simulink model "HANcoder_E407_Matrix"  (R2018b)
settings: Solver=FixedStepDiscrete  StartTime=0.0  StopTime=1  FixedStep=0.01  RelTol=1e-3
PreLoadFcn:
  | librarySetup
  | eval([bdroot,'_startup']) %Calling [modelName]_startup.m
undefined symbols (not defined in the file): frequency_IRQ, HANtuneOverride, idle_time, LED_ticks_toggle
libraries: HANcoder_STM32_Target x15, simulink x6, simulink_extras x1
CloseFcn:
  | rtwprivate ssgencode ModelCloseRequest mytest
settings Model: Creator=Jason van Kolfschoten  LastModifiedBy=Jamie
settings SolverCC: PositivePriorityOrder=on
settings DataIOCC: LimitDataPoints=on  SaveFormat=Array  SignalLoggingSaveFormat=ModelDataLogs  SaveOutput=off  SaveTime=off
settings OptimizationCC: BlockReduction=off  DefaultParameterBehavior=Inlined  InlineInvariantSignals=on  ExpressionDepthLimit=2147483647  StateBitsets=on  DataBitsets=on  ZeroExternalMemoryAtStartup=off  ZeroInternalMemoryAtStartup=off  InitFltsAndDblsToZero=on  NoFixptDivByZeroProtection=on  EfficientFloat2IntCast=on  LifeSpan=inf
settings DebuggingCC: SaveWithDisabledLinksMsg=none  SaveWithParameterizedLinksMsg=none  CheckSSInitialOutputMsg=off  UnderspecifiedInitializationDetection=Classic  MergeDetectMultiDrivingBlocksExec=none  SignalResolutionControl=TryResolveAll  SolverPrmCheckMsg=warning  InheritedTsInSrcMsg=none  MultiTaskDSMMsg=warning  MultiTaskCondExecSysMsg=none  ParameterPrecisionLossMsg=none  FcnCallInpInsideContextMsg=warning  StateNameClashWarn=warning  SFUnexpectedBacktrackingDiag=warning  SFNoUnconditionalDefaultTransitionDiag=warning  SFExecutionAtInitializationDiag=none
settings HardwareCC: ProdBitPerPointer=32  ProdBitPerSizeT=32  ProdBitPerPtrDiffT=32  ProdLargestAtomicFloat=None  ProdIntDivRoundTo=Undefined  ProdWordSize=32  ProdHWDeviceType=Generic->32-bit Embedded Processor  TargetEndianess=LittleEndian  TargetHWDeviceType=Infineon->TriCore
settings ModelReferenceCC: PropagateSignalLabelsOutOfModel=off
settings SFSimCC: SimUseLocalCustomCode=off  MATLABDynamicMemAlloc=off
settings RTWCC: SystemTargetFile=ert.tlc  MakeCommand=make_rtw SHELL= HANcoder_PORTABLE=1 HANcoder_BOOTLOADER=1  TemplateMakefile=STM32_E407_gcc.tmf  Description=Real-Time Workshop Embedded Coder (no auto configuration)  RTWUseLocalCustomCode=off
settings CodeAppCC: ForceParamTrailComments=on  IgnoreCustomStorageClasses=off  SimulinkDataObjDesc=on  CustomSymbolStrGlobalVar=rt$N$M  CustomSymbolStrType=$N$M  CustomSymbolStrFcn=$N$M$F  CustomSymbolStrMacro=$N$M  InsertBlockDesc=on  StateflowObjectComments=on  InternalIdentifier=Classic
settings ERTTargetCC: TargetFcnLib=ansi_tfl_tmw.mat  MultiwordLength=2048  IncludeMdlTerminateFcn=off  SuppressErrorStatus=on  SupportNonFinite=off  GenerateASAP2=on  InlinedParameterPlacement=NonHierarchical  ERTCustomFileTemplate=example_file_process.tlc  ConvertIfToSwitch=off  SuppressUnreachableDefaultCases=off
settings ConfigComp: CovMetricSettings=dw  CovHtmlReporting=on  CovSaveCumulativeToWorkspaceVar=on  CovSaveSingleToWorkspaceVar=on  CovExternalEMLEnable=off  DVMaxProcessTime=600  DVDisplayUnsatisfiableObjectives=on  DVAutomaticStubbing=off  DVModelCoverageObjectives=MCDC  DVMaxTestCaseSteps=500  DVTestSuiteOptimization=CombinedObjectives  DVDetectActiveLogic=on  DVSaveHarnessModel=on

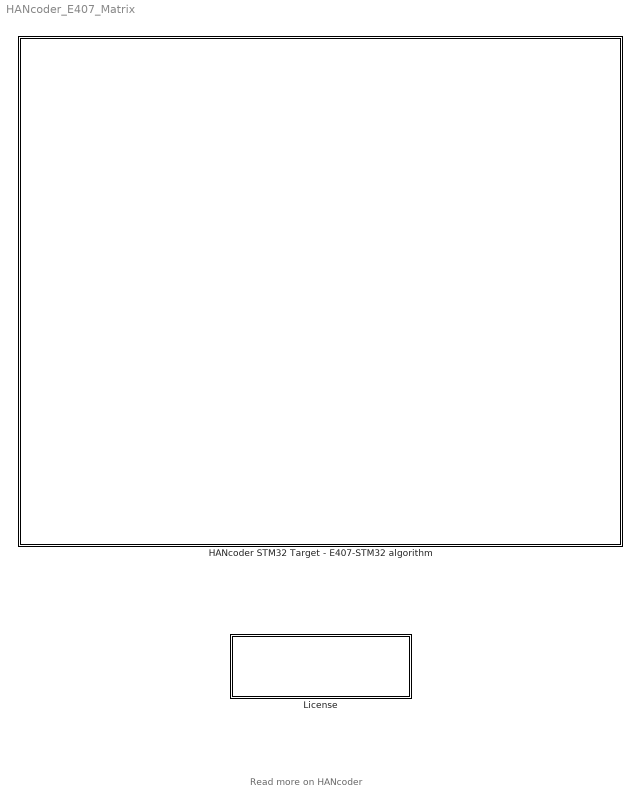
== system HANcoder_E407_Matrix ==
  note: Read more on HANcoder
  HANcoder STM32 Target - E407-STM32 algorithm : Subsystem  mask(TopLevelSubsystem){}
      settings: CopyFcn=HANcoderChecks('Copy');  NameChangeFcn=HANcoderChecks('NameChangeE407');  MoveFcn=HANcoderChecks('MoveE407');
      mask Display: image(imread('STM32_E407_HAN.jpg'))
  License : Subsystem  mask(License){}
      settings: NameChangeFcn=HANcoderChecks('NameChangeLicenseBlock');  OpenFcn=winopen('License.pdf')  MoveFcn=HANcoderChecks('MoveLicenseBlock');
      mask Display: disp(['End-User License Agreement\n','please read before use']);

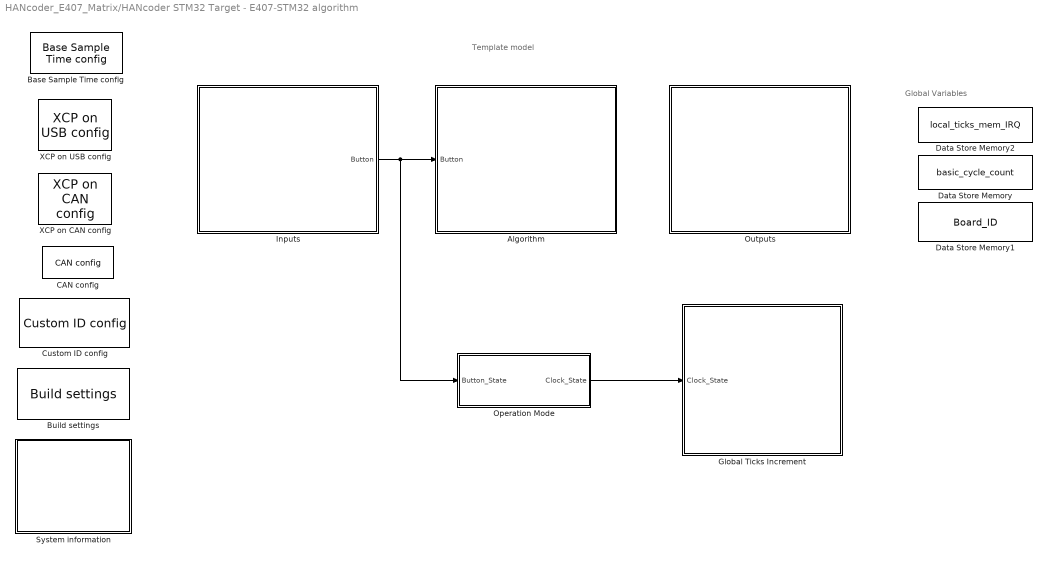
== system HANcoder_E407_Matrix/HANcoder STM32 Target - E407-STM32 algorithm ==
  note: Template model
  note: Global Variables
  Algorithm : Subsystem
  Base Sample Time config : HANcoder_STM32_Target/STM32-E407/System Config/Base Sample Time config  Tag=HANcoder_TARGET_STM32_E407  Description=HANcoder Target STM32-E407 blockset version 0.5  baseSampleTime=10  extraStack=0
      settings: SourceProductName=HANcoder STM32 Target
  Build settings : HANcoder_STM32_Target/STM32-E407/System Config/Build settings  Tag=HANcoder_TARGET_STM32_E407  AutoASAP2add=on  AutoFlash=USB
      settings: SourceProductName=HANcoder STM32 Target
  CAN config : HANcoder_STM32_Target/STM32-E407/System Config/CAN config  Tag=HANcoder_TARGET_STM32_E407  txBufSize=64  evBufSize=8  canBus1=off  baudRate1=500  rxMask1=hex2dec('00000000')  rxCode1=hex2dec('00000000')  rxMode1=Receive only 11-bit message identifiers  canBus2=on  baudRate2=500  rxMask2=hex2dec('00000000')  rxCode2=hex2dec('00000000')  rxMode2=Receive only 11-bit message identifiers
      settings: SourceProductName=HANcoder STM32 Target
  Custom ID config : HANcoder_STM32_Target/STM32-E407/System Config/Custom ID config  Tag=HANcoder_TARGET_STM32_E407  softID=softwareID  softNUM=1
      settings: SourceProductName=HANcoder STM32 Target
  Data Store Memory : DataStoreMemory  DataStoreName=basic_cycle_count  ReadBeforeWriteMsg=warning  WriteAfterWriteMsg=warning  WriteAfterReadMsg=warning  ShowAdditionalParam=off  OutDataTypeStr=uint8
  Data Store Memory1 : DataStoreMemory  DataStoreName=Board_ID  ReadBeforeWriteMsg=warning  WriteAfterWriteMsg=warning  WriteAfterReadMsg=warning  ShowAdditionalParam=off
  Data Store Memory2 : DataStoreMemory  DataStoreName=local_ticks_mem_IRQ  ReadBeforeWriteMsg=warning  WriteAfterWriteMsg=warning  WriteAfterReadMsg=warning  ShowAdditionalParam=off  OutDataTypeStr=uint32
  Global Ticks Increment : Subsystem
  Inputs : Subsystem
  Operation Mode : Subsystem
  Outputs : Subsystem
  System information : Subsystem
  XCP on CAN config : HANcoder_STM32_Target/STM32-E407/System Config/XCP on CAN config  Tag=HANcoder_TARGET_STM32_E407  canBus=CAN 2  croID=hex2dec('665')  dtoID=hex2dec('666')
      settings: SourceProductName=HANcoder STM32 Target
  XCP on USB config : HANcoder_STM32_Target/STM32-E407/System Config/XCP on USB config  Tag=HANcoder_TARGET_STM32_E407
      settings: SourceProductName=HANcoder STM32 Target
  wires:
  Operation Mode/1(Clock_State) -> Global Ticks Increment/1(Clock_State)
  Inputs/1(Button) -> Operation Mode/1(Button_State), Algorithm/1(Button)

== system HANcoder_E407_Matrix/License ==

== system HANcoder_E407_Matrix/HANcoder STM32 Target - E407-STM32 algorithm/Algorithm ==
  note: The button or the HANtuneOverride parameter
      | switches between the two frequencies.
  note: Here the algorithm can be placed. No hardware dependent blocks should be used here.
  note: Switch LED frequency when button is pressed
  Button : Inport
  10Hz Counter Limiter : simulink/Sources/Counter Limited  uplimit=1  tsamp=0.1
  5Hz Counter Limited : simulink/Sources/Counter Limited  uplimit=1  tsamp=0.2
  Constant : Constant  Value=HANtuneOverride  OutDataTypeStr=boolean
  Data Type Conversion : DataTypeConversion  OutDataTypeStr=boolean
  Logical Operator : Logic  Operator=OR  AllPortsSameDT=off  OutDataTypeStr=boolean
  Switch : Switch  Criteria=u2 > Threshold
  Terminator : Terminator
  wires:
  Data Type Conversion/1 -> Terminator/1  "LedValue"
  5Hz Counter Limited/1 -> Switch/3
  Switch/1 -> Data Type Conversion/1
  Button/1 -> Logical Operator/2
  Logical Operator/1 -> Switch/2
  Constant/1 -> Logical Operator/1
  10Hz Counter Limiter/1 -> Switch/1

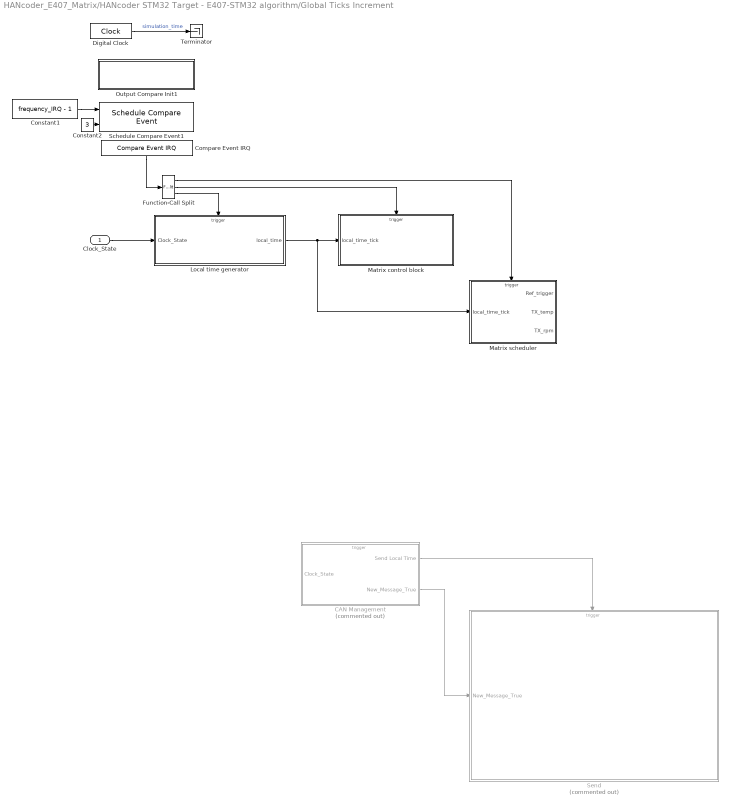
== system HANcoder_E407_Matrix/HANcoder STM32 Target - E407-STM32 algorithm/Global Ticks Increment ==
  Clock_State : Inport
  CAN Management : Subsystem  Commented=on
  Compare Event IRQ : HANcoder_STM32_Target/STM32-E407/Timer Outputs/Compare Event IRQ  Tag=HANcoder_TARGET_STM32_E407  pin=TIM4 - CON PD - 15 - 5V Tolerant
      settings: SourceProductName=HANcoder STM32 Target
  Constant1 : Constant  Value=frequency_IRQ - 1  OutDataTypeStr=uint16
  Constant2 : Constant  Value=3  OutDataTypeStr=uint8
  Digital Clock : DigitalClock  SampleTime=0.01
  Function-Call Split : FunctionCallSplit  IconShape=distinctive  NumOutputPorts=3  OutputPortLayout=default
  Local time generator : Subsystem  TreatAsAtomicUnit=on
  Matrix control block : Subsystem  TreatAsAtomicUnit=on
  Matrix scheduler : Subsystem  TreatAsAtomicUnit=on
  Output Compare Init1 : Subsystem  Tag=HANcoder_TARGET_STM32_E407  AncestorBlock=HANcoder_STM32_Target/STM32-E407/Timer Outputs/Output Compare Init  mask(Output Compare Init){moduleID=TIM4 - CON PD - 15 & 16 &n/a & n/a, frequency=1000000, enableIRQoutput=off}
      mask prompts: moduleID "Timer module"; frequency "Frequency (free running counter) [Hz]"; enableIRQoutput "Enable IRQ output"
      mask help:
      | Function
      | ========
      | Initializes the timer module to allow output compare functionality on the
      | module's channels.
      |
      | Parameters
      | ==========
      | Timer Module:
      |   Selects the timer module.
      |
      | Frequency:
      |   Frequency at which the 16-bit free running counter counts.
      |
      | Enable IRQ output
      |   Controls whether or not the IRQ output is available.
      |
      | Outport
      | =======
      | IRQ
      |   Allows connection of a function call subsystem for the free running
      |   counter overflow event.
      mask init:
      | moduleIDInfoStr = sfcn_timeout_init_mcb(2, moduleID, frequency, enableIRQoutput);
      settings: CopyFcn=sfcn_timeout_init_chk();  MoveFcn=drawLogos
      mask Help: web('sfcn_timeout_init.html');
      mask TypeOptions moduleID: TIM1 - CON PE - 12 & 14 & 16 & 17 | TIM2 - CON4 - D13 & n/a & n/a & n/a | TIM3 - CON4 - D12 & D11 & n/a & n/a | TIM4 - CON PD - 15 & 16 &n/a & n/a | TIM8 - UEXT - 3 & 4 & n/a & n/a | TIM9 - CON3 - D4 & D5 or PE - 8 & 9 | TIM10 - CON2 - A1 or CON PF - 9 | TIM11 - CON2 - A2 or CON PF - 10 | TIM13 - CON2 - A3 or CON PF - 11 | TIM14 - CON2 - A4 or CON PF - 12
      mask Callback moduleID: sfcn_timeout_init_chk();
      mask Display: fprintf('Output Compare Init\n%s', moduleIDInfoStr);patch([135 141 141],[8 14 2],[1 0 0]);patch([143 143 149],[14 2 8],[0 0 0.35]);
  Schedule Compare Event1 : HANcoder_STM32_Target/STM32-E407/Timer Outputs/Schedule Compare Event  Tag=HANcoder_TARGET_STM32_E407  pin=TIM4 - CON PD - 15 - 5V Tolerant  tsamp=-1
      settings: SourceProductName=HANcoder STM32 Target
  Send : Subsystem  Commented=on
  Terminator : Terminator
  wires:
  Clock_State/1 -> Local time generator/1(Clock_State)
  Digital Clock/1 -> Terminator/1  "simulation_time"
  Constant2/1 -> Schedule Compare Event1/2
  Constant1/1 -> Schedule Compare Event1/1
  CAN Management/1(Send Local Time) -> Send/Trigger
  CAN Management/2(New_Message_True) -> Send/1(New_Message_True)
  Local time generator/1("local_time ") -> Matrix scheduler/1(local_time_tick), Matrix control block/1(local_time_tick)
  Compare Event IRQ/1 -> Function-Call Split/1
  Function-Call Split/3 -> Local time generator/Trigger
  Function-Call Split/2 -> Matrix control block/Trigger
  Function-Call Split/1 -> Matrix scheduler/Trigger

== system HANcoder_E407_Matrix/HANcoder STM32 Target - E407-STM32 algorithm/Inputs ==
  note: The inputs and outputs are kept in a separate subsystem, this way the algorithm can easily be transferred to different hardware
  Digital Input : HANcoder_STM32_Target/STM32-E407/Digital Inputs/Digital Input  Tag=HANcoder_TARGET_STM32_E407  pinID=WKUP button  config=Pulldown  tsamp=-1
      settings: SourceProductName=HANcoder STM32 Target
  Button : Outport
  wires:
  Digital Input/1 -> Button/1

== system HANcoder_E407_Matrix/HANcoder STM32 Target - E407-STM32 algorithm/Operation Mode ==
  note: Operation Mode
      | There are two modes of operation:
      | ( 0 ) Idle (Clock Off)
      | ( 1 ) Counting (Clock On)
      | In order to switch from one to the other the Olimexino button
      | must be pressed once. In this subsystem, with every negative
      | edge of the Button State, the Operation Mode will change from
      | one to the other.
  Button_State : Inport
  Constant : Constant  OutDataTypeStr=boolean
  Flip Flop T : Subsystem
  Clock_State : Outport
  wires:
  Constant/1 -> Flip Flop T/1(T)
  Button_State/1 -> Flip Flop T/2(Clk)
  Flip Flop T/1(Q) -> Clock_State/1

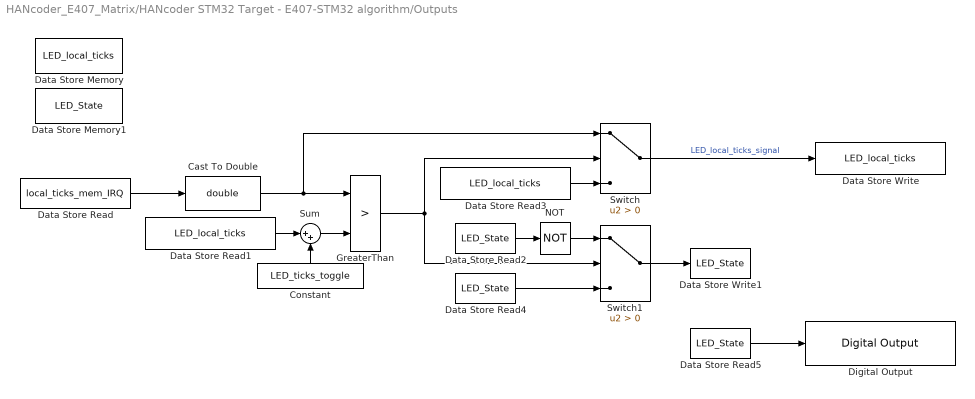
== system HANcoder_E407_Matrix/HANcoder STM32 Target - E407-STM32 algorithm/Outputs ==
  Cast To Double : DataTypeConversion  OutDataTypeStr=double
  Constant : Constant  Value=LED_ticks_toggle
  Data Store Memory : DataStoreMemory  DataStoreName=LED_local_ticks  ReadBeforeWriteMsg=warning  WriteAfterWriteMsg=warning  WriteAfterReadMsg=warning  ShowAdditionalParam=off
  Data Store Memory1 : DataStoreMemory  DataStoreName=LED_State  ReadBeforeWriteMsg=warning  WriteAfterWriteMsg=warning  WriteAfterReadMsg=warning  ShowAdditionalParam=off  OutDataTypeStr=boolean
  Data Store Read : DataStoreRead  DataStoreName=local_ticks_mem_IRQ
  Data Store Read1 : DataStoreRead  DataStoreName=LED_local_ticks
  Data Store Read2 : DataStoreRead  DataStoreName=LED_State
  Data Store Read3 : DataStoreRead  DataStoreName=LED_local_ticks
  Data Store Read4 : DataStoreRead  DataStoreName=LED_State
  Data Store Read5 : DataStoreRead  DataStoreName=LED_State
  Data Store Write : DataStoreWrite  DataStoreName=LED_local_ticks
  Data Store Write1 : DataStoreWrite  DataStoreName=LED_State
  Digital Output : HANcoder_STM32_Target/STM32-E407/Digital Outputs/Digital Output  Tag=HANcoder_TARGET_STM32_E407  pinID=LED  config=Push pull  tsamp=-1
      settings: SourceProductName=HANcoder STM32 Target
  GreaterThan : RelationalOperator  Operator=>  OutDataTypeStr=boolean  RndMeth=Simplest
  NOT : Logic  Operator=NOT  IconShape=distinctive  AllPortsSameDT=off  OutDataTypeStr=boolean
  Sum : Sum  Inputs=|++
  Switch : Switch  Criteria=u2 > Threshold
  Switch1 : Switch  Criteria=u2 > Threshold
  wires:
  Data Store Read1/1 -> Sum/1
  Sum/1 -> GreaterThan/2
  Constant/1 -> Sum/2
  GreaterThan/1 -> Switch/2, Switch1/2
  Switch/1 -> Data Store Write/1  "LED_local_ticks_signal"
  Data Store Read/1 -> Cast To Double/1
  Data Store Read3/1 -> Switch/3
  Cast To Double/1 -> GreaterThan/1, Switch/1
  Switch1/1 -> Data Store Write1/1
  Data Store Read2/1 -> NOT/1
  NOT/1 -> Switch1/1
  Data Store Read4/1 -> Switch1/3
  Data Store Read5/1 -> Digital Output/1

== system HANcoder_E407_Matrix/HANcoder STM32 Target - E407-STM32 algorithm/System information ==
  note: These blocks check the free memory: stack and heap and the CPU load,
      | this way you can see whether your software demands too much of the microcontroller
  Get CPU load : HANcoder_STM32_Target/STM32-E407/System Management/Get CPU load  Tag=HANcoder_TARGET_STM32_E407  mode=Current CPU load  tsamp=-1
      settings: SourceProductName=HANcoder STM32 Target
  Get free Heap : HANcoder_STM32_Target/STM32-E407/System Management/Get free Heap  Tag=HANcoder_TARGET_STM32_E407  tsamp=-1
      settings: SourceProductName=HANcoder STM32 Target
  Get free Stack : HANcoder_STM32_Target/STM32-E407/System Management/Get free Stack  Tag=HANcoder_TARGET_STM32_E407  taskIdx=Application Control Task  tsamp=-1
      settings: SourceProductName=HANcoder STM32 Target
  Terminator : Terminator
  Terminator1 : Terminator
  Terminator2 : Terminator
  wires:
  Get CPU load/1 -> Terminator1/1  "SI_CPUload"
  Get free Stack/1 -> Terminator/1  "SI_FreeStack"
  Get free Heap/1 -> Terminator2/1  "SI_FreeHeap"

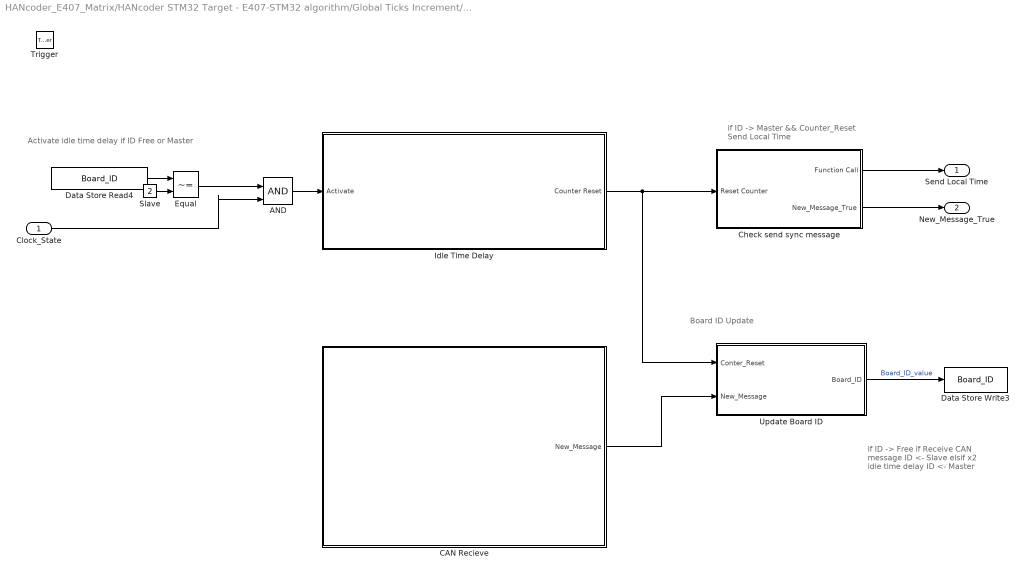
== system HANcoder_E407_Matrix/HANcoder STM32 Target - E407-STM32 algorithm/Global Ticks Increment/CAN Management ==
  note: Activate idle time delay if ID
      |    Free or Master
  note: Board ID Update
  note: if ID -> Master && Counter_Reset
      | 	Send Local Time
  note: if ID -> Free
      | 	if Receive CAN message
      | 		ID <- Slave
      | 	elsif x2 idle time delay
      | 		ID <- Master
  Clock_State : Inport
  Trigger : TriggerPort  TriggerType=function-call  VariantControl=Variant  PortDimensions=1
  AND : Logic  IconShape=distinctive  AllPortsSameDT=off  OutDataTypeStr=boolean
  CAN Recieve : Subsystem
  Check send sync message : Subsystem
  Data Store Read4 : DataStoreRead  DataStoreName=Board_ID
  Data Store Write3 : DataStoreWrite  DataStoreName=Board_ID
  Equal : RelationalOperator  Operator=~=  OutDataTypeStr=boolean  RndMeth=Simplest
  Idle Time Delay : Subsystem
  Slave : Constant  Value=2
  Update Board ID : Subsystem
  Send Local Time : Outport
  New_Message_True : Outport  Port=2
  wires:
  Data Store Read4/1 -> Equal/1
  Equal/1 -> AND/1
  Slave/1 -> Equal/2
  Idle Time Delay/1(Counter Reset) -> Check send sync message/1(Reset Counter), Update Board ID/1(Conter_Reset)
  CAN Recieve/1(New_Message) -> Update Board ID/2(New_Message)
  Update Board ID/1(Board_ID) -> Data Store Write3/1  "Board_ID_value"
  Check send sync message/1(Function Call) -> Send Local Time/1
  Clock_State/1 -> AND/2
  AND/1 -> Idle Time Delay/1(Activate)
  Check send sync message/2(New_Message_True) -> New_Message_True/1

== system HANcoder_E407_Matrix/HANcoder STM32 Target - E407-STM32 algorithm/Global Ticks Increment/Local time generator ==
  note: Counter Reset
  note: Tick Counter Increment
  Clock_State : Inport
  function : TriggerPort  TriggerType=function-call  VariantControl=Variant
  Constant : Constant  OutDataTypeStr=uint32
  Data Store Read : DataStoreRead  DataStoreName=local_ticks_mem_IRQ
  Data Store Read1 : DataStoreRead  DataStoreName=local_ticks_mem_IRQ
  Data Store Write : DataStoreWrite  DataStoreName=local_ticks_mem_IRQ
  Even_Tick : Stateflow chart  TreatAsAtomicUnit=on
  Odd_Tick : Stateflow chart  TreatAsAtomicUnit=on
  Reset Free Running Counter1 : HANcoder_STM32_Target/STM32-E407/Timer Outputs/Reset Free Running Counter  Tag=HANcoder_TARGET_STM32_E407  moduleID=TIM4 - CON PD - 15 & 16 &n/a & n/a
      settings: SourceProductName=HANcoder STM32 Target
  Reset Free Running Counter2 : HANcoder_STM32_Target/STM32-E407/Timer Outputs/Reset Free Running Counter  Tag=HANcoder_TARGET_STM32_E407  moduleID=TIM4 - CON PD - 15 & 16 &n/a & n/a
      settings: SourceProductName=HANcoder STM32 Target
  Sum : Sum
  Switch : Switch  Criteria=u2 > Threshold
  "local_time " : Outport
  wires:
  Constant/1 -> Sum/2
  Switch/1 -> Data Store Write/1, Even_Tick/1(current_tick), Odd_Tick/1(current_tick)  "local_ticks_interrupt"
  Clock_State/1 -> Switch/2
  Data Store Read/1 -> "local_time "/1, Sum/1
  Sum/1 -> Switch/1
  Data Store Read1/1 -> Switch/3
  Even_Tick/1(rise_edge_at_even) -> Reset Free Running Counter1/Trigger  "even"
  Odd_Tick/1(rise_edge_at_odd) -> Reset Free Running Counter2/Trigger  "odd"

== system HANcoder_E407_Matrix/HANcoder STM32 Target - E407-STM32 algorithm/Global Ticks Increment/Matrix control block ==
  local_time_tick : Inport
  function : TriggerPort  TriggerType=function-call  VariantControl=Variant
  Reset values : Subsystem  TreatAsAtomicUnit=on
  True if end of basic cycle : If  IfExpression=u1 == cycle_duration  ShowElse=off
  wires:
  local_time_tick/1 -> True if end of basic cycle/1
  True if end of basic cycle/1 -> Reset values/Action

== system HANcoder_E407_Matrix/HANcoder STM32 Target - E407-STM32 algorithm/Global Ticks Increment/Matrix scheduler ==
  note: Reference message (Master only)
  note: TX triggers
  local_time_tick : Inport
  function : TriggerPort  TriggerType=function-call  VariantControl=Variant
  AND : Logic  IconShape=distinctive  AllPortsSameDT=off  OutDataTypeStr=boolean
  Compare To Constant : simulink/Logic and Bit Operations/Compare To Constant  relop===  const=0  OutDataTypeStr=boolean
  Compare To Constant1 : simulink/Logic and Bit Operations/Compare To Constant  relop===  const=1  OutDataTypeStr=boolean
  Compare To Constant2 : simulink/Logic and Bit Operations/Compare To Constant  relop===  const=25000  OutDataTypeStr=boolean
  Compare To Constant3 : simulink/Logic and Bit Operations/Compare To Constant  relop===  const=50000  OutDataTypeStr=boolean
  Data Store Read4 : DataStoreRead  DataStoreName=Board_ID
  Ref_trigger : Outport
  TX_temp : Outport  Port=2
  TX_rpm : Outport  Port=3
  wires:
  Data Store Read4/1 -> Compare To Constant1/1
  Compare To Constant3/1 -> TX_rpm/1
  AND/1 -> Ref_trigger/1
  local_time_tick/1 -> Compare To Constant/1, Compare To Constant3/1, Compare To Constant2/1
  Compare To Constant1/1 -> AND/2
  Compare To Constant2/1 -> TX_temp/1
  Compare To Constant/1 -> AND/1

== system HANcoder_E407_Matrix/HANcoder STM32 Target - E407-STM32 algorithm/Global Ticks Increment/Output Compare Init1 ==
  S-Function : S-Function  FunctionName=sfcn_timeout_init  SFunctionDeploymentMode=off  EnableBusSupport=off
  Term1 : Terminator
  wires:
  S-Function/1 -> Term1/1

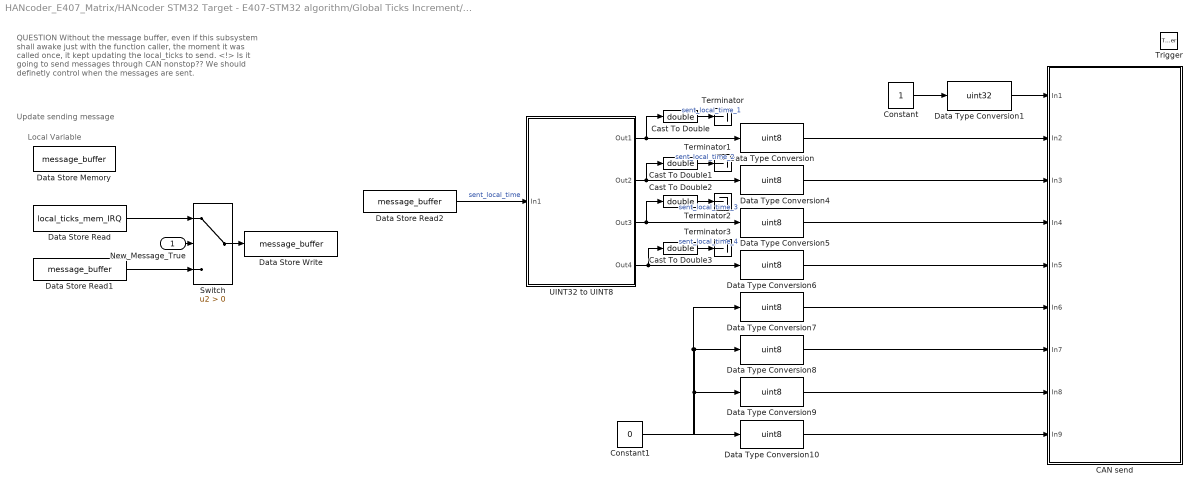
== system HANcoder_E407_Matrix/HANcoder STM32 Target - E407-STM32 algorithm/Global Ticks Increment/Send ==
  note: QUESTION
      | Without the message buffer, even if this subsystem shall
      | awake just with the function caller, the moment it was called
      | once, it kept updating the local_ticks to send.
      | <!> Is it going to send messages through CAN nonstop??
      | We should definetly control when the messages are sent.
  note: Update sending message
  note: Local Variable
  New_Message_True : Inport
  Trigger : TriggerPort  TriggerType=function-call  VariantControl=Variant  PortDimensions=1
  CAN send : Subsystem  Tag=HANcoder_TARGET_STM32_E407  AncestorBlock=HANcoder_STM32_Target/STM32-E407/CAN/CAN/CAN send  mask(CAN send){canBus=CAN 2, frameType=Standard (11 bit), inputNumber=8, dataType=uint8, byteOrder=off, tsamp=-1}
      mask prompts: canBus "CAN channel"; frameType "Identifier type"; inputNumber "Input ports"; dataType "Input datatype"; byteOrder "Byte order: Checked = MSB first, unchecked = LSB first."; tsamp "Sample time"
      mask help:
      | Function
      | ==========
      | Send a message on the CAN channel.
      |
      | Parameters
      | ==========
      | CAN channel:           The CAN channel to send the message on.
      | Identifier type:         normal or extended ID's
      | Input ports:              The amount of input ports
      | Input datatype:        The datatype of the input ports
      | Byte order:               Select MSB or LSB first
      | Sample time:            -1 or divisible by base sample time [seconds]
      |
      | Input
      | ==========
      | Port 1:                   CAN ID(uint32) in hexadecimal ie: hex2dec('0a')
      | Port 2..9                CAN message data
      mask init:
      | sfcn_can_send_mcb(canBus, frameType, inputNumber, dataType, byteOrder)
      settings: MoveFcn=drawLogos
      mask Help: web('sfcn_can_send.html');
      mask TypeOptions canBus: CAN 1 | CAN 2
      mask TypeOptions frameType: Standard (11 bit) | Extended (29 bit)
      mask TypeOptions dataType: int8 | uint8 | int16 | uint16 | int32 | uint32 | boolean
      mask Display:
      | fprintf('Send on\nCAN %x', canBus);
      | port_label('input', 1, 'ID');patch([140 146 146],[8 14 2],[1 0 0]);patch([148 148 154],[14 2 8],[0 0 0.35]);
  Cast To Double{,1..3} (4 alike) : DataTypeConversion  OutDataTypeStr=double
  Constant : Constant
  Constant1 : Constant  Value=0
  Data Store Memory : DataStoreMemory  DataStoreName=message_buffer  ReadBeforeWriteMsg=warning  WriteAfterWriteMsg=warning  WriteAfterReadMsg=warning  ShowAdditionalParam=off  OutDataTypeStr=uint32
  Data Store Read : DataStoreRead  DataStoreName=local_ticks_mem_IRQ
  Data Store Read1 : DataStoreRead  DataStoreName=message_buffer
  Data Store Read2 : DataStoreRead  DataStoreName=message_buffer
  Data Store Write : DataStoreWrite  DataStoreName=message_buffer
  Data Type Conversion{,4..10} (8 alike) : DataTypeConversion  OutDataTypeStr=uint8
  Data Type Conversion1 : DataTypeConversion  OutDataTypeStr=uint32
  Switch : Switch  Criteria=u2 > Threshold
  Terminator{,1..3} (4 alike) : Terminator
  UINT32 to UINT8 : Subsystem
  wires:
  Data Type Conversion10/1 -> CAN send/9(In9)
  Data Type Conversion/1 -> CAN send/2(In2)
  Data Type Conversion1/1 -> CAN send/1(In1)
  Data Type Conversion9/1 -> CAN send/8(In8)
  Data Type Conversion8/1 -> CAN send/7(In7)
  Constant/1 -> Data Type Conversion1/1
  Data Type Conversion5/1 -> CAN send/4(In4)
  Data Type Conversion4/1 -> CAN send/3(In3)
  Data Type Conversion6/1 -> CAN send/5(In5)
  Data Type Conversion7/1 -> CAN send/6(In6)
  Constant1/1 -> Data Type Conversion7/1, Data Type Conversion10/1, Data Type Conversion9/1, Data Type Conversion8/1
  UINT32 to UINT8/1(Out1) -> Cast To Double/1, Data Type Conversion/1
  UINT32 to UINT8/2(Out2) -> Cast To Double1/1, Data Type Conversion4/1
  UINT32 to UINT8/3(Out3) -> Cast To Double2/1, Data Type Conversion5/1
  UINT32 to UINT8/4(Out4) -> Cast To Double3/1, Data Type Conversion6/1
  Cast To Double/1 -> Terminator/1  "sent_local_time_1"
  Cast To Double1/1 -> Terminator1/1  "sent_local_time_2"
  Cast To Double2/1 -> Terminator2/1  "sent_local_time_3"
  Cast To Double3/1 -> Terminator3/1  "sent_local_time_4"
  Data Store Read/1 -> Switch/1
  New_Message_True/1 -> Switch/2
  Data Store Read1/1 -> Switch/3
  Switch/1 -> Data Store Write/1
  Data Store Read2/1 -> UINT32 to UINT8/1(In1)  "sent_local_time"

== system HANcoder_E407_Matrix/HANcoder STM32 Target - E407-STM32 algorithm/Operation Mode/Flip Flop T ==
  T : Inport  OutDataTypeStr=boolean
  Clk : Inport  Port=2  OutDataTypeStr=boolean
  J-K Flip-Flop : simulink_extras/Flip Flops/J-K Flip-Flop  initial_condition=0
      settings: SourceProductName=Simulink
  Terminator : Terminator
  Q : Outport  OutDataTypeStr=boolean
  wires:
  J-K Flip-Flop/2 -> Terminator/1
  T/1 -> J-K Flip-Flop/3, J-K Flip-Flop/1
  J-K Flip-Flop/1 -> Q/1
  Clk/1 -> J-K Flip-Flop/2

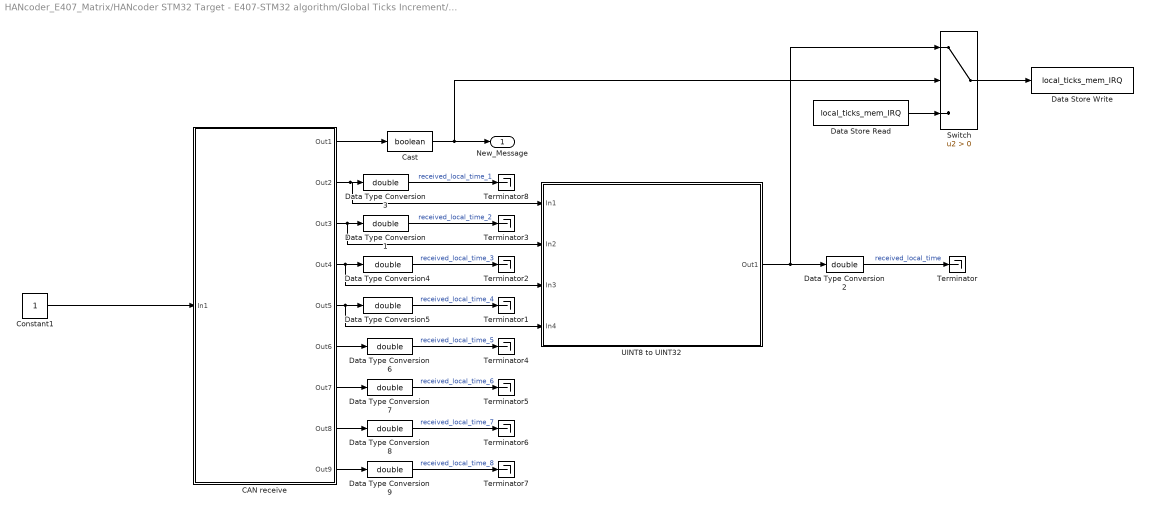
== system HANcoder_E407_Matrix/HANcoder STM32 Target - E407-STM32 algorithm/Global Ticks Increment/CAN Management/CAN Recieve ==
  CAN receive : Subsystem  Tag=HANcoder_TARGET_STM32_E407  AncestorBlock=HANcoder_STM32_Target/STM32-E407/CAN/CAN/CAN receive  mask(CAN receive){canBus=CAN 2, outputNumber=8, dataType=uint8, byteOrder=off, tsamp=-1}
      mask prompts: canBus "CAN channel"; outputNumber "Output ports"; dataType "Output datatype"; byteOrder "Byte order: Checked = MSB first, unchecked = LSB first."; tsamp "Sample time"
      mask help:
      | Function
      | ==========
      | Receive the newest message from the specified CAN channel.
      |
      | Parameters
      | ==========
      | CAN channel:             The CAN channel to send the message on.
      | Output ports:             The amount of output ports
      | Output datatype:       The datatype of the output ports
      | Byte order:                 Select MSB or LSB first
      | Sample time:              -1 or divisible by base sample time [seconds]
      |
      | Input
      | ==========
      | Port 1:                       CAN ID(uint32) in hexadecimal ie: hex2dec('0a')
      |
      | Output
      | ==========
      | Port 1:                       Checks for new message(int8)
      | Port 2..9                     Message data
      mask init:
      | sfcn_can_receive_mcb(canBus, outputNumber, dataType, byteOrder)
      settings: MoveFcn=drawLogos
      mask Help: web('sfcn_can_receive.html');
      mask TypeOptions canBus: CAN 1 | CAN 2
      mask TypeOptions dataType: int8 | uint8 | int16 | uint16 | int32 | uint32 | boolean
      mask Display:
      | fprintf('Receive on\nCAN %x', canBus);
      | port_label('output', 1, 'new');
      | port_label('input', 1, 'ID');patch([155 161 161],[8 14 2],[1 0 0]);patch([163 163 169],[14 2 8],[0 0 0.35]);
  Cast : DataTypeConversion  OutDataTypeStr=boolean
  Constant1 : Constant  OutDataTypeStr=uint32
  Data Store Read : DataStoreRead  DataStoreName=local_ticks_mem_IRQ
  Data Store Write : DataStoreWrite  DataStoreName=local_ticks_mem_IRQ
  Data Type Conversion{1..9} (9 alike) : DataTypeConversion  OutDataTypeStr=double
  Switch : Switch  Criteria=u2 > Threshold
  Terminator{,1..8} (9 alike) : Terminator
  UINT8 to UINT32 : Subsystem
  New_Message : Outport
  wires:
  CAN receive/9(Out9) -> Data Type Conversion9/1
  CAN receive/6(Out6) -> Data Type Conversion6/1
  Data Type Conversion7/1 -> Terminator5/1  "received_local_time_6"
  CAN receive/4(Out4) -> UINT8 to UINT32/3(In3), Data Type Conversion4/1
  CAN receive/8(Out8) -> Data Type Conversion8/1
  Data Type Conversion5/1 -> Terminator1/1  "received_local_time_4"
  Constant1/1 -> CAN receive/1(In1)
  CAN receive/1(Out1) -> Cast/1
  Data Type Conversion4/1 -> Terminator2/1  "received_local_time_3"
  Data Type Conversion1/1 -> Terminator3/1  "received_local_time_2"
  CAN receive/3(Out3) -> UINT8 to UINT32/2(In2), Data Type Conversion1/1
  Data Type Conversion3/1 -> Terminator8/1  "received_local_time_1"
  Data Type Conversion8/1 -> Terminator6/1  "received_local_time_7"
  Data Type Conversion9/1 -> Terminator7/1  "received_local_time_8"
  CAN receive/5(Out5) -> UINT8 to UINT32/4(In4), Data Type Conversion5/1
  CAN receive/2(Out2) -> UINT8 to UINT32/1(In1), Data Type Conversion3/1
  Data Type Conversion6/1 -> Terminator4/1  "received_local_time_5"
  CAN receive/7(Out7) -> Data Type Conversion7/1
  UINT8 to UINT32/1(Out1) -> Switch/1, Data Type Conversion2/1
  Data Type Conversion2/1 -> Terminator/1  "received_local_time"
  Cast/1 -> New_Message/1, Switch/2
  Data Store Read/1 -> Switch/3
  Switch/1 -> Data Store Write/1

== system HANcoder_E407_Matrix/HANcoder STM32 Target - E407-STM32 algorithm/Global Ticks Increment/CAN Management/Check send sync message ==
  note: Activate Master sync message
  note: Send sync message if ID
      |    Master
  Reset Counter : Inport
  AND : Logic  IconShape=distinctive  AllPortsSameDT=off  OutDataTypeStr=boolean
  Check_Reset_Idle_Time : Stateflow chart  TreatAsAtomicUnit=on
  Data Store Read2 : DataStoreRead  DataStoreName=Board_ID
  Equal1 : RelationalOperator  Operator===  OutDataTypeStr=boolean  RndMeth=Simplest
  Master : Constant
  Function Call : Outport
  New_Message_True : Outport  Port=2
  wires:
  AND/1 -> New_Message_True/1, Check_Reset_Idle_Time/1(reset_idle_counter)
  Data Store Read2/1 -> Equal1/1
  Master/1 -> Equal1/2
  Check_Reset_Idle_Time/1(send_local_time()) -> Function Call/1
  Equal1/1 -> AND/1
  Reset Counter/1 -> AND/2

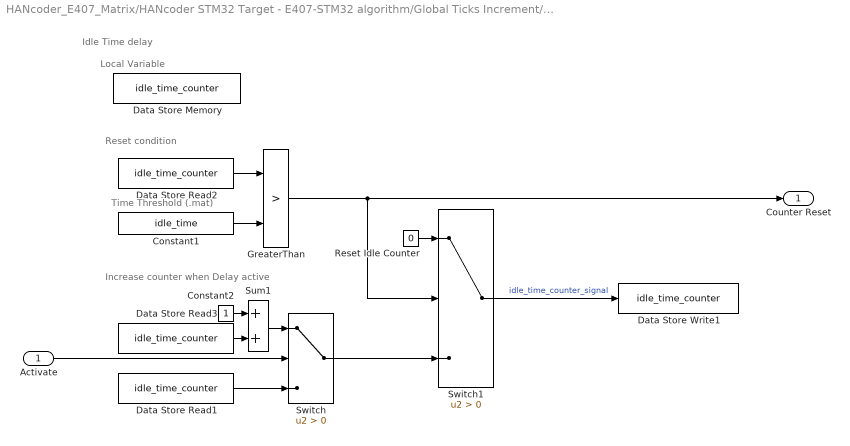
== system HANcoder_E407_Matrix/HANcoder STM32 Target - E407-STM32 algorithm/Global Ticks Increment/CAN Management/Idle Time Delay ==
  note: Time Threshold (.mat)
  note: Increase counter when Delay active
  note: Reset condition
  note: Idle Time delay
  note: Local Variable
  Activate : Inport
  Constant1 : Constant  Value=idle_time
  Constant2 : Constant
  Data Store Memory : DataStoreMemory  DataStoreName=idle_time_counter  ReadBeforeWriteMsg=warning  WriteAfterWriteMsg=warning  WriteAfterReadMsg=warning  ShowAdditionalParam=off
  Data Store Read1 : DataStoreRead  DataStoreName=idle_time_counter
  Data Store Read2 : DataStoreRead  DataStoreName=idle_time_counter
  Data Store Read3 : DataStoreRead  DataStoreName=idle_time_counter
  Data Store Write1 : DataStoreWrite  DataStoreName=idle_time_counter
  GreaterThan : RelationalOperator  Operator=>  OutDataTypeStr=boolean  RndMeth=Simplest
  Reset Idle Counter : Constant  Value=0
  Sum1 : Sum
  Switch : Switch  Criteria=u2 > Threshold
  Switch1 : Switch  Criteria=u2 > Threshold
  Counter Reset : Outport
  wires:
  Constant2/1 -> Sum1/1
  GreaterThan/1 -> Switch1/2, Counter Reset/1
  Data Store Read2/1 -> GreaterThan/1
  Constant1/1 -> GreaterThan/2
  Reset Idle Counter/1 -> Switch1/1
  Switch1/1 -> Data Store Write1/1  "idle_time_counter_signal"
  Data Store Read3/1 -> Sum1/2
  Sum1/1 -> Switch/1
  Activate/1 -> Switch/2
  Data Store Read1/1 -> Switch/3
  Switch/1 -> Switch1/3

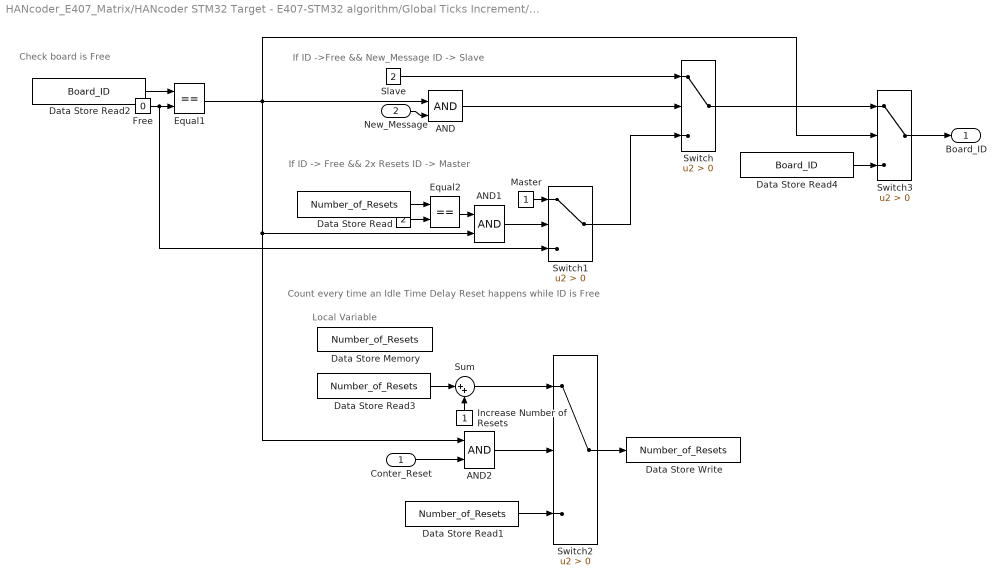
== system HANcoder_E407_Matrix/HANcoder STM32 Target - E407-STM32 algorithm/Global Ticks Increment/CAN Management/Update Board ID ==
  note: Count every time an Idle Time Delay Reset happens while ID is Free
  note: Local Variable
  note: If ID -> Free && 2x Resets
      |    ID -> Master
  note: If ID ->Free && New_Message
      |    ID -> Slave
  note: Check board is Free
  Conter_Reset : Inport
  New_Message : Inport  Port=2
  " " : Constant  Value=2
  AND : Logic  IconShape=distinctive  AllPortsSameDT=off  OutDataTypeStr=boolean
  AND1 : Logic  IconShape=distinctive  AllPortsSameDT=off  OutDataTypeStr=boolean
  AND2 : Logic  IconShape=distinctive  AllPortsSameDT=off  OutDataTypeStr=boolean
  Data Store Memory : DataStoreMemory  DataStoreName=Number_of_Resets  ReadBeforeWriteMsg=warning  WriteAfterWriteMsg=warning  WriteAfterReadMsg=warning  ShowAdditionalParam=off
  Data Store Read : DataStoreRead  DataStoreName=Number_of_Resets
  Data Store Read1 : DataStoreRead  DataStoreName=Number_of_Resets
  Data Store Read2 : DataStoreRead  DataStoreName=Board_ID
  Data Store Read3 : DataStoreRead  DataStoreName=Number_of_Resets
  Data Store Read4 : DataStoreRead  DataStoreName=Board_ID
  Data Store Write : DataStoreWrite  DataStoreName=Number_of_Resets
  Equal1 : RelationalOperator  Operator===  OutDataTypeStr=boolean  RndMeth=Simplest
  Equal2 : RelationalOperator  Operator===  OutDataTypeStr=boolean  RndMeth=Simplest
  Free : Constant  Value=0
  Increase Number of Resets : Constant
  Master : Constant
  Slave : Constant  Value=2
  Sum : Sum  Inputs=|++
  Switch{,1..3} (4 alike) : Switch  Criteria=u2 > Threshold
  Board_ID : Outport
  wires:
  Switch/1 -> Switch3/1
  Data Store Read2/1 -> Equal1/1
  Free/1 -> Switch1/3, Equal1/2
  Equal1/1 -> Switch3/2, AND2/1, AND1/2, AND/1
  New_Message/1 -> AND/2
  AND/1 -> Switch/2
  Slave/1 -> Switch/1
  Master/1 -> Switch1/1
  Switch1/1 -> Switch/3
  Data Store Read/1 -> Equal2/1
  Switch2/1 -> Data Store Write/1
  Conter_Reset/1 -> AND2/2
  Data Store Read1/1 -> Switch2/3
  Data Store Read3/1 -> Sum/1
  Increase Number of Resets/1 -> Sum/2
  Sum/1 -> Switch2/1
  AND1/1 -> Switch1/2
  " "/1 -> Equal2/2
  Equal2/1 -> AND1/1
  AND2/1 -> Switch2/2
  Switch3/1 -> Board_ID/1
  Data Store Read4/1 -> Switch3/3

== system HANcoder_E407_Matrix/HANcoder STM32 Target - E407-STM32 algorithm/Global Ticks Increment/Matrix control block/Reset values ==
  note: Basic cycle counter
  Action Port : ActionPort  ActionType=then
  Add : Sum
  Constant1 : Constant  Value=0  OutDataTypeStr=uint32
  Constant2 : Constant  OutDataTypeStr=uint8
  Data Store Read : DataStoreRead  DataStoreName=basic_cycle_count
  Data Store Read1 : DataStoreRead  DataStoreName=basic_cycle_count
  Data Store Write : DataStoreWrite  DataStoreName=local_ticks_mem_IRQ
  Data Store Write2 : DataStoreWrite  DataStoreName=basic_cycle_count
  If : If  IfExpression=u1 == matrix_rows  ShowElse=off
  If Action Subsystem : Subsystem  TreatAsAtomicUnit=on
  wires:
  Constant1/1 -> Data Store Write/1
  Data Store Read/1 -> If/1
  If/1 -> If Action Subsystem/Action
  Data Store Read1/1 -> Add/1
  Constant2/1 -> Add/2
  Add/1 -> Data Store Write2/1  "bc"

== system HANcoder_E407_Matrix/HANcoder STM32 Target - E407-STM32 algorithm/Global Ticks Increment/Send/CAN send ==
  In1 : Inport
  In2 : Inport  Port=2
  In3 : Inport  Port=3
  In4 : Inport  Port=4
  In5 : Inport  Port=5
  In6 : Inport  Port=6
  In7 : Inport  Port=7
  In8 : Inport  Port=8
  In9 : Inport  Port=9
  S-Function : M-S-Function  FunctionName=sfcn_can_send  Parameters=tsamp, canBus, frameType, inputNumber, dataType, byteOrder
  wires:
  In1/1 -> S-Function/1
  In2/1 -> S-Function/2
  In3/1 -> S-Function/3
  In4/1 -> S-Function/4
  In5/1 -> S-Function/5
  In6/1 -> S-Function/6
  In7/1 -> S-Function/7
  In8/1 -> S-Function/8
  In9/1 -> S-Function/9

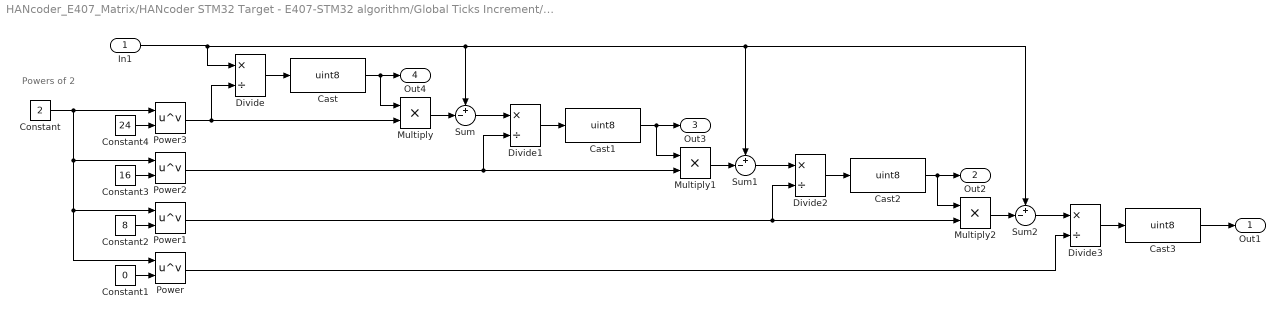
== system HANcoder_E407_Matrix/HANcoder STM32 Target - E407-STM32 algorithm/Global Ticks Increment/Send/UINT32 to UINT8 ==
  note: Powers of 2
  In1 : Inport
  Cast{,1..3} (4 alike) : DataTypeConversion  OutDataTypeStr=uint8
  Constant : Constant  Value=2
  Constant1 : Constant  Value=0
  Constant2 : Constant  Value=8
  Constant3 : Constant  Value=16
  Constant4 : Constant  Value=24
  Divide{,1..3} (4 alike) : Product  Inputs=*/
  Multiply : Product
  Multiply1 : Product
  Multiply2 : Product
  Power{,1..3} (4 alike) : Math  Operator=pow  SaturateOnIntegerOverflow=on
  Sum : Sum  Inputs=+-|
  Sum1 : Sum  Inputs=+-|
  Sum2 : Sum  Inputs=+-|
  Out1 : Outport
  Out2 : Outport  Port=2
  Out3 : Outport  Port=3
  Out4 : Outport  Port=4
  wires:
  Constant2/1 -> Power1/2
  Constant3/1 -> Power2/2
  Constant4/1 -> Power3/2
  Power2/1 -> Multiply1/2, Divide1/2
  Constant1/1 -> Power/2
  Power3/1 -> Divide/2, Multiply/2
  Constant/1 -> Power/1, Power1/1, Power2/1, Power3/1
  Divide/1 -> Cast/1
  Cast/1 -> Multiply/1, Out4/1
  Multiply/1 -> Sum/2
  Divide1/1 -> Cast1/1
  Sum/1 -> Divide1/1
  Cast1/1 -> Out3/1, Multiply1/1
  Multiply1/1 -> Sum1/2
  Multiply2/1 -> Sum2/2
  Cast2/1 -> Out2/1, Multiply2/1
  Divide2/1 -> Cast2/1
  Power1/1 -> Multiply2/2, Divide2/2
  Sum1/1 -> Divide2/1
  Sum2/1 -> Divide3/1
  In1/1 -> Sum1/1, Sum2/1, Sum/1, Divide/1
  Power/1 -> Divide3/2
  Divide3/1 -> Cast3/1
  Cast3/1 -> Out1/1

== system HANcoder_E407_Matrix/HANcoder STM32 Target - E407-STM32 algorithm/Global Ticks Increment/CAN Management/CAN Recieve/CAN receive ==
  In1 : Inport
  Enabled Subsystem : Subsystem  TreatAsAtomicUnit=on
  S-Function : M-S-Function  FunctionName=sfcn_can_receive  Parameters=tsamp, canBus, outputNumber, dataType, byteOrder
  Out1 : Outport
  Out2 : Outport  Port=2
  Out3 : Outport  Port=3
  Out4 : Outport  Port=4
  Out5 : Outport  Port=5
  Out6 : Outport  Port=6
  Out7 : Outport  Port=7
  Out8 : Outport  Port=8
  Out9 : Outport  Port=9
  wires:
  S-Function/9 -> Enabled Subsystem/8(In8)
  S-Function/4 -> Enabled Subsystem/3(In3)
  S-Function/5 -> Enabled Subsystem/4(In4)
  S-Function/8 -> Enabled Subsystem/7(In7)
  S-Function/7 -> Enabled Subsystem/6(In6)
  S-Function/6 -> Enabled Subsystem/5(In5)
  Enabled Subsystem/8(Out8) -> Out9/1
  Enabled Subsystem/7(Out7) -> Out8/1
  Enabled Subsystem/6(Out6) -> Out7/1
  Enabled Subsystem/5(Out5) -> Out6/1
  Enabled Subsystem/4(Out4) -> Out5/1
  Enabled Subsystem/3(Out3) -> Out4/1
  Enabled Subsystem/2(Out2) -> Out3/1
  Enabled Subsystem/1(Out1) -> Out2/1
  S-Function/3 -> Enabled Subsystem/2(In2)
  S-Function/2 -> Enabled Subsystem/1(In1)
  S-Function/1 -> Out1/1, Enabled Subsystem/Enable
  In1/1 -> S-Function/1

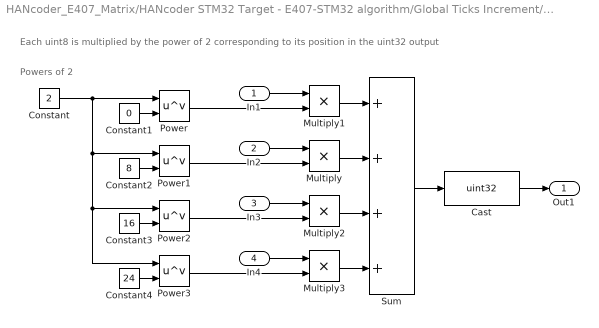
== system HANcoder_E407_Matrix/HANcoder STM32 Target - E407-STM32 algorithm/Global Ticks Increment/CAN Management/CAN Recieve/UINT8 to UINT32 ==
  note: Each uint8 is multiplied by the power of 2 corresponding to its position in the uint32 output
  note: Powers of 2
  In1 : Inport
  In2 : Inport  Port=2
  In3 : Inport  Port=3
  In4 : Inport  Port=4
  Cast : DataTypeConversion  OutDataTypeStr=uint32
  Constant : Constant  Value=2
  Constant1 : Constant  Value=0
  Constant2 : Constant  Value=8
  Constant3 : Constant  Value=16
  Constant4 : Constant  Value=24
  Multiply{,1..3} (4 alike) : Product
  Power{,1..3} (4 alike) : Math  Operator=pow  SaturateOnIntegerOverflow=on
  Sum : Sum  Inputs=++++
  Out1 : Outport
  wires:
  Cast/1 -> Out1/1
  Sum/1 -> Cast/1
  In1/1 -> Multiply1/1
  In2/1 -> Multiply/1
  In3/1 -> Multiply2/1
  In4/1 -> Multiply3/1
  Constant/1 -> Power3/1, Power2/1, Power1/1, Power/1
  Constant1/1 -> Power/2
  Constant2/1 -> Power1/2
  Constant3/1 -> Power2/2
  Constant4/1 -> Power3/2
  Power/1 -> Multiply1/2
  Power1/1 -> Multiply/2
  Power2/1 -> Multiply2/2
  Power3/1 -> Multiply3/2
  Multiply3/1 -> Sum/4
  Multiply2/1 -> Sum/3
  Multiply/1 -> Sum/2
  Multiply1/1 -> Sum/1

== system HANcoder_E407_Matrix/HANcoder STM32 Target - E407-STM32 algorithm/Global Ticks Increment/Matrix control block/Reset values/If Action Subsystem ==
  Action Port : ActionPort  ActionType=then
  Constant : Constant  Value=0  OutDataTypeStr=uint8
  Data Store Write1 : DataStoreWrite  DataStoreName=basic_cycle_count
  wires:
  Constant/1 -> Data Store Write1/1

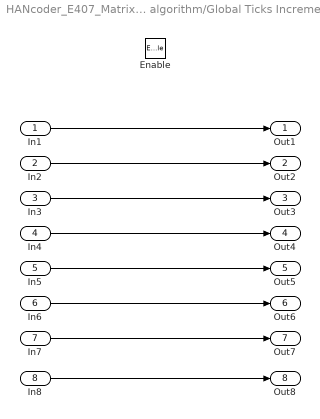
== system HANcoder_E407_Matrix/HANcoder STM32 Target - E407-STM32 algorithm/Global Ticks Increment/CAN Management/CAN Recieve/CAN receive/Enabled Subsystem ==
  In1 : Inport
  In2 : Inport  Port=2
  In3 : Inport  Port=3
  In4 : Inport  Port=4
  In5 : Inport  Port=5
  In6 : Inport  Port=6
  In7 : Inport  Port=7
  In8 : Inport  Port=8
  Enable : EnablePort
  Out1 : Outport
  Out2 : Outport  Port=2
  Out3 : Outport  Port=3
  Out4 : Outport  Port=4
  Out5 : Outport  Port=5
  Out6 : Outport  Port=6
  Out7 : Outport  Port=7
  Out8 : Outport  Port=8
  wires:
  In8/1 -> Out8/1
  In7/1 -> Out7/1
  In6/1 -> Out6/1
  In5/1 -> Out5/1
  In4/1 -> Out4/1
  In3/1 -> Out3/1
  In2/1 -> Out2/1
  In1/1 -> Out1/1

== stateflow chart HANcoder_E407_Matrix/HANcoder STM32 Target - E407-STM32 algorithm/Global Ticks Increment/Local time generator/Even_Tick ==
  settings: initializeOutput=1
  state Even_tick
    if (mod(current_tick,2)==0)
    active_flag = 1;
    end
  state Rise_edge
    send(rise_edge_at_even)
  (default) -> Even_tick
  Even_tick -> Rise_edge : [active_flag == 1]
  data: current_tick input; active_flag local =0
  events: rise_edge_at_even output EITHER_EDGE_EVENT

== stateflow chart HANcoder_E407_Matrix/HANcoder STM32 Target - E407-STM32 algorithm/Global Ticks Increment/CAN Management/Check send sync message/Check_Reset_Idle_Time ==
  settings: initializeOutput=1
  state Check_Reset
    if reset_idle_counter
    active_flag = 1;
    else
    active_flag = 0;
    end
  state Reset_True
    send(send_local_time)
  (default) -> Check_Reset
  Check_Reset -> Reset_True : [active_flag == 1]
  data: reset_idle_counter input; active_flag local =0
  events: send_local_time output FUNCTION_CALL_EVENT

== stateflow chart HANcoder_E407_Matrix/HANcoder STM32 Target - E407-STM32 algorithm/Global Ticks Increment/Local time generator/Odd_Tick ==
  settings: initializeOutput=1
  state Odd_tick
    if (mod(current_tick,2)==1)
    active_flag = 1;
    end
  state Rise_edge
    send(rise_edge_at_odd)
  (default) -> Odd_tick
  Odd_tick -> Rise_edge : [active_flag == 1]
  data: current_tick input; active_flag local =0
  events: rise_edge_at_odd output EITHER_EDGE_EVENT
